simulink model "model_for_testing_errors_2"  (R2023b)
settings: Solver=VariableStepAuto  StartTime=0.0  StopTime=time_model  FixedStep=0.0001  RelTol=1e-3
values from neighbouring files (symbols this model uses):
  A_flap = [c_a, c_b, 0 ... (first row only)    [LQR_calculate.m]    (also in LQR_feedback.m; LQR_linearized_test.m; MPC_test.m; MPC_test_1.m)
  A_ind = [c_d, 0, 0 ... (first row only)    [LQR_calculate.m]    (also in LQR_feedback.m; LQR_linearized_test.m; MPC_test.m; MPC_test_1.m)
  C_drag = 0    [LQR_calculate.m]    (also in LQR_feedback.m = C_drag_arr(i); LQR_linearized_test.m = C_drag_arr(i); MPC_test.m = C_drag_arr(i); MPC_test_1.m = C_drag_arr(i))
  demp = 0    [LQR_feedback.m]    (also in LQR_linearized_test.m; MPC_params.m; MPC_test_1.m; initQuadrotorData.m)
  forward_1 = 20    [LQR_feedback.m]    (also in LQR_linearized_test.m; MPC_test_1.m)
  forward_2 = 20    [LQR_feedback.m]    (also in LQR_linearized_test.m; MPC_test_1.m)
  g = 9.81    [LQR_calculate.m]    (also in LQR_feedback.m = 9.8; LQR_linearized_test.m = 9.8; LQR_testing_gpt.m; MPC_params.m = 9.8)
  Im = 0.0135^2*0.045/2    (= 4.100625e-06)    [LQR_calculate.m]    (also in LQR_feedback.m; LQR_linearized_test.m; MPC_params.m; MPC_test.m)
  Ix = m/3*a^2/12+2*0.045*l^2    (= 0.00211347222222)    [LQR_calculate.m]    (also in LQR_feedback.m; LQR_linearized_test.m; LQR_testing_gpt.m = 0.0081; MPC_params.m)
  Iy = m/3*a^2/12+4*0.045*l^2    (= 0.00413847222222)    [LQR_calculate.m]    (also in LQR_feedback.m = 0.00211347222222; LQR_linearized_test.m = 0.00211347222222; LQR_testing_gpt.m = 0.0081; MPC_params.m = 0.00211347222222)
  Iz = m/3*a^2/4+2*0.045*l^2    (= 0.00229041666667)    [LQR_calculate.m]    (also in LQR_feedback.m = 0.00431541666667; LQR_linearized_test.m = 0.00431541666667; LQR_testing_gpt.m = 0.0142; MPC_params.m = 0.00431541666667)
  J = 2.5*10^(-6)    (= 2.5e-06)    [LQR_calculate.m]    (also in LQR_feedback.m; LQR_linearized_test.m; MPC_params.m; MPC_test.m)
  K = Y * inv(P)    [LQR_calculate.m]    (also in LQR_feedback.m = [Kx;Ky;Kz;Kphi;Ktheta;-Kpsi])
  Ke = ke    (= 0.0073)    [LQR_calculate.m]    (also in LQR_feedback.m = 0.00734; LQR_linearized_test.m = 0.00734; MPC_params.m = 0.00734; MPC_test.m)
  kf = ks*r^2*airDensity*Sblade/2    (= 1.57565625e-05)    [LQR_calculate.m]    (also in LQR_feedback.m; LQR_linearized_test.m; MPC_params.m; MPC_test.m)
  Km = kt    (= 0.0073)    [LQR_calculate.m]    (also in LQR_feedback.m = 0.00734; LQR_linearized_test.m = 0.00734; MPC_params.m = 0.00734; MPC_test.m)
  kv = 1300    [LQR_feedback.m]    (also in LQR_linearized_test.m; MPC_test_1.m; initQuadrotorData.m)
  l = 0.15    [LQR_calculate.m]    (also in LQR_feedback.m; LQR_linearized_test.m; MPC_params.m; MPC_test.m)
  L = La    (= 5e-05)    [LQR_calculate.m]    (also in LQR_feedback.m = 0.0001; LQR_linearized_test.m = 0.0001; MPC_params.m = 0.0001; MPC_test.m)
  m = size(B, 2)    [LQR_calculate.m]    (also in LQR_feedback.m = 0.65; LQR_linearized_test.m = 0.65; LQR_testing_gpt.m = 1; MPC_params.m = 0.65)
  Mode = 3    [LQR_feedback.m]    (also in LQR_linearized_test.m; MPC_test_1.m = 1)
  phi0 = 0    [LQR_feedback.m]    (also in LQR_linearized_test.m; MPC_test_1.m)
  psi0 = pi/2    (= 1.57079632679)    [LQR_feedback.m]    (also in LQR_linearized_test.m; MPC_test_1.m = 0)
  Psid = 0    [LQR_feedback.m]    (also in LQR_linearized_test.m; MPC_test_1.m)
  R = eye(4)    [LQR_calculate.m]    (also in LQR_feedback.m = 0.058; LQR_linearized_test.m = 0.058; LQR_testing_gpt.m = diag([0.1, 10, 100, 10]); MPC_params.m = 0.058)
  rho = 1.225    [LQR_calculate.m]    (also in LQR_feedback.m; LQR_linearized_test.m; MPC_params.m; MPC_test.m)
  S = l*c*4+a*b    (= 0.0169)    [LQR_calculate.m]    (also in LQR_feedback.m; LQR_linearized_test.m; MPC_params.m; MPC_test.m)
  theta0 = 0    [LQR_feedback.m]    (also in LQR_linearized_test.m; MPC_test_1.m)
  time_model = time_model_arr(i)    [LQR_feedback.m]    (also in LQR_linearized_test.m; MPC_test.m; MPC_test_1.m; plot_model_out.m)
  total_time = 60    [LQR_feedback.m]    (also in LQR_linearized_test.m; MPC_test_1.m)
  up_down = 5    [LQR_feedback.m]    (also in LQR_linearized_test.m; MPC_test_1.m)
  x0 = 0    [LQR_feedback.m]    (also in LQR_linearized_test.m; MPC_test_1.m; init_nmpc.m = zeros(nx,1))
  Xd = [Simulation.trajectory.Data(1,:)',Simulation.trajectory.Data(2,:)',Simulation.trajectory.Data(3,:)',Simulation.trajectory.Data(9,:)']    [LQR_feedback.m]    (also in LQR_linearized_test.m; MPC_test_1.m; plot_model_out.m)
  y0 = 0    [LQR_feedback.m]    (also in LQR_linearized_test.m; MPC_test_1.m)
  Yd = 0    [LQR_feedback.m]    (also in LQR_linearized_test.m; MPC_test_1.m)
  z0 = 0    [LQR_feedback.m]    (also in LQR_linearized_test.m; MPC_test_1.m)
  Zd = 0    [LQR_feedback.m]    (also in LQR_linearized_test.m; MPC_test_1.m)
libraries: sharedtransform x1
(part 1 of 2)
settings Model: Creator=Degra  LastModifiedBy=Degra

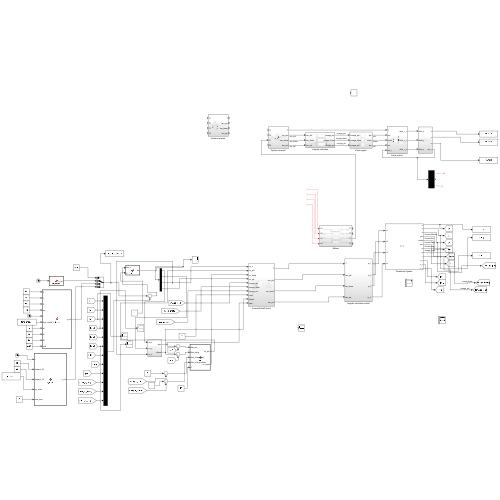
[thumbnail: Simulink's stored preview of the top-level diagram]
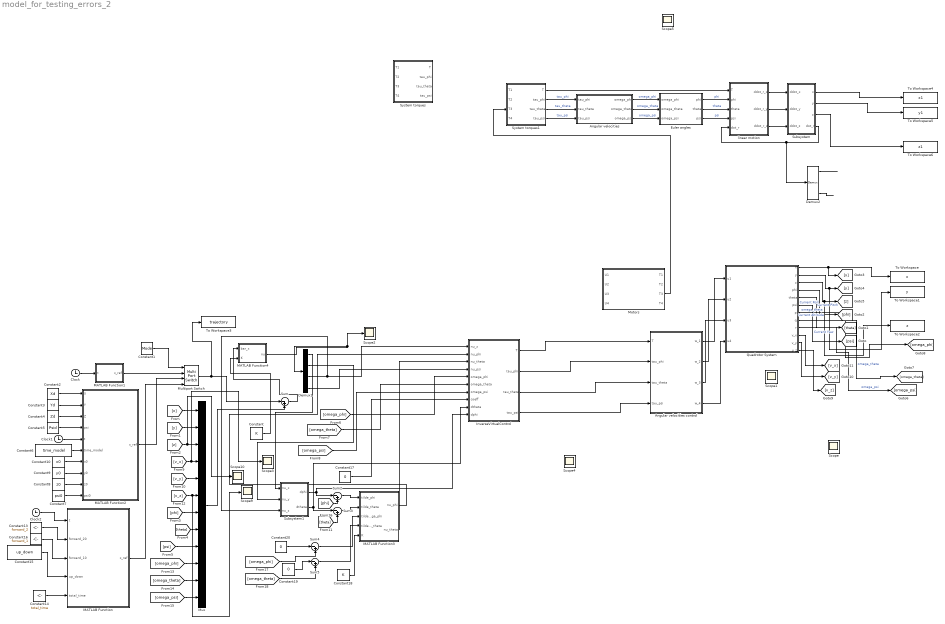
== system model_for_testing_errors_2 ==
  Angular velocities : Subsystem
  Angular velocities control : Subsystem
  Clock : Clock
  Clock1 : Clock
  Clock2 : Clock
  Constant : Constant  Value=K
  Constant1 : Constant  Value=Mode
  Constant10 : Constant  Value=x0
  Constant13 : Constant  Value=forward_2
  Constant14 : Constant  Value=total_time
  Constant15 : Constant  Value=up_down
  Constant16 : Constant  Value=forward_1
  Constant17 : Constant  Value=0
  Constant18 : Constant  Value=K
  Constant19 : Constant  Value=0
  Constant2 : Constant  Value=Xd
  Constant20 : Constant  Value=0
  Constant3 : Constant  Value=Yd
  Constant4 : Constant  Value=Zd
  Constant5 : Constant  Value=Psid
  Constant6 : Constant  Value=time_model
  Constant7 : Constant  Value=psi0
  Constant8 : Constant  Value=z0
  Constant9 : Constant  Value=y0
  Demux1 : Demux
  Demux2 : Demux  Outputs=3
  Euler angles : Subsystem
  InverseVirtualControl : Subsystem
  MATLAB Function : MATLAB Function  TreatAsAtomicUnit=on
  MATLAB Function1 : MATLAB Function  TreatAsAtomicUnit=on
  MATLAB Function2 : MATLAB Function  TreatAsAtomicUnit=on
  MATLAB Function3 : MATLAB Function  TreatAsAtomicUnit=on
  MATLAB Function4 : MATLAB Function  TreatAsAtomicUnit=on
  Motors : Subsystem
  Multiport Switch : MultiPortSwitch  SaturateOnIntegerOverflow=off  InputSameDT=off
  Mux : Mux  Inputs=12
  Quadrotor System : Subsystem
      mask Display: image('C:\Users\angel\OneDrive - Universidad Politécnica de Yucatán\CIMAT\1st semester\Robotic Systems Modeling and Control\Project\Quadrotor\images\quadrotor.jpg');
  Scope : Scope  NumInputPorts=4
  Scope1 : Scope  NumInputPorts=4
  Scope{2..5,9..10} (6 alike) : Scope
  Subsystem : Subsystem
  Subsystem1 : Subsystem
  Sum{,2..5} (5 alike) : Sum  Inputs=|-+
  System torques : Subsystem
  System torques1 : Subsystem
  To Workspace : ToWorkspace  VariableName=x  SaveFormat=Timeseries  SampleTime=-1
  To Workspace1 : ToWorkspace  VariableName=y  SaveFormat=Timeseries  SampleTime=-1
  To Workspace2 : ToWorkspace  VariableName=z  SaveFormat=Timeseries  SampleTime=-1
  To Workspace3 : ToWorkspace  VariableName=trajectory  SaveFormat=Timeseries  SampleTime=-1
  To Workspace4 : ToWorkspace  VariableName=x1  SaveFormat=Timeseries  SampleTime=-1
  To Workspace5 : ToWorkspace  VariableName=y1  SaveFormat=Timeseries  SampleTime=-1
  To Workspace6 : ToWorkspace  VariableName=z1  SaveFormat=Timeseries  SampleTime=-1
  linear motion : Subsystem
  wires:
  Quadrotor System/1(x) -> To Workspace/1, [x]
  Quadrotor System/2(y) -> To Workspace1/1, [y]
  Quadrotor System/3(z) -> To Workspace2/1, [z]  "Current Altitude"
  Quadrotor System/6(psi) -> [psi]  "Current Yaw"
  Quadrotor System/5(theta) -> [theta]  "Current Pitch"
  Quadrotor System/4(phi) -> [phi]  "Current Roll"
  Quadrotor System/9(r) -> [omega_psi]  "omega_psi"
  Quadrotor System/8(q) -> [omega_theta]  "omega_theta"
  Quadrotor System/7(p) -> [omega_phi]  "omega_theta"
  Quadrotor System/10(v_x) -> [v_x]
  Quadrotor System/11(v_y) -> [v_y]
  Quadrotor System/12(v_z) -> [v_z]
  ? -> Motors/4(U4)
  ? -> Motors/3(U3)
  ? -> Motors/2(U2)
  ? -> Motors/1(U1)
  Motors/3(T3) -> System torques1/3(T3)
  Demux2/1 -> ?
  linear motion/1(ddot_r_x) -> Subsystem/1(ddot_x)
  Demux2/3 -> ?
  Angular velocities/1(omega_phi) -> Euler angles/1(omega_phi)  "omega_phi"
  linear motion/2(ddot_r_y) -> Subsystem/2(ddot_y)
  linear motion/3(ddot_r_z) -> Subsystem/3(ddot_z)
  Euler angles/2(theta) -> linear motion/3(theta)  "theta"
  Euler angles/3(psi) -> linear motion/4(psi)  "psi"
  Euler angles/1(phi) -> linear motion/2(phi)  "phi"
  Angular velocities/2(omega_theta) -> Euler angles/2(omega_theta)  "omega_theta"
  Angular velocities/3(omega_psi) -> Euler angles/3(omega_psi)  "omega_psi"
  Subsystem/4(dot_r) -> Demux2/1, linear motion/5(dot_r)
  Subsystem/2(y) -> To Workspace5/1
  Subsystem/1(x) -> To Workspace4/1
  Subsystem/3(z) -> To Workspace6/1
  System torques1/4(tau_psi) -> Angular velocities/3(tau_psi)  "tau_psi"
  System torques1/3(tau_theta) -> Angular velocities/2(tau_theta)  "tau_theta"
  System torques1/2(tau_phi) -> Angular velocities/1(tau_phi)  "tau_phi"
  System torques1/1(T) -> linear motion/1(T)
  [omega_phi] -> Sum4/2
  MATLAB Function3/2(nu_theta) -> InverseVirtualControl/3(nu_theta)
  InverseVirtualControl/1(T) -> Angular velocities control/1(T)
  Subsystem1/1(dphi) -> Sum2/1, InverseVirtualControl/10(dphi)
  Sum4/1 -> MATLAB Function3/3(tilde_omega_phi)
  MATLAB Function3/1(nu_phi) -> InverseVirtualControl/2(nu_phi)
  Sum2/1 -> MATLAB Function3/1(tilde_phi)
  Demux1/4 -> InverseVirtualControl/4(nu_psi)
  Constant18/1 -> MATLAB Function3/5(K)
  [omega_theta] -> Sum5/2
  [phi] -> Sum2/2
  Sum5/1 -> MATLAB Function3/4(tilde_omega_theta)
  [theta] -> Sum3/2
  Sum3/1 -> MATLAB Function3/2(tilde_theta)
  [omega_theta] -> InverseVirtualControl/6(omega_theta)
  [omega_psi] -> InverseVirtualControl/7(omega_psi)
  Constant1/1 -> Multiport Switch/1
  Demux1/1 -> Subsystem1/1(nu_x)
  Constant/1 -> MATLAB Function4/2(K)
  InverseVirtualControl/4(tau_psi) -> Angular velocities control/4("tau_psi ")
  MATLAB Function4/1(nu) -> Scope2/1, Demux1/1
  Constant17/1 -> InverseVirtualControl/8(coeff)
  Sum/1 -> MATLAB Function4/1(bar_x)
  [phi] -> Mux/7
  Constant9/1 -> MATLAB Function2/8(y0)
  Constant6/1 -> MATLAB Function2/6(time_model)
  [omega_phi] -> InverseVirtualControl/5(omega_phi)
  MATLAB Function2/1(x_ref) -> Multiport Switch/3
  Constant20/1 -> Sum4/1
  InverseVirtualControl/2(tau_phi) -> Angular velocities control/2(tau_phi)
  Clock1/1 -> MATLAB Function2/5(t)
  Constant7/1 -> MATLAB Function2/10(psi0)
  Clock2/1 -> MATLAB Function/1(t)
  Demux1/3 -> Subsystem1/3(nu_z), InverseVirtualControl/1(nu_z)
  Constant19/1 -> Sum5/1
  [omega_theta] -> Mux/11
  Constant15/1 -> MATLAB Function/4(up_down)
  Constant16/1 -> MATLAB Function/3(forward_10)
  Constant13/1 -> MATLAB Function/2(forward_20)
  Subsystem1/2(dtheta) -> Sum3/1, InverseVirtualControl/9(dtheta)
  MATLAB Function1/1(x_ref) -> Multiport Switch/2
  Constant14/1 -> MATLAB Function/5(total_time)
  Mux/1 -> Sum/2
  Constant10/1 -> MATLAB Function2/7(x0)
  [omega_psi] -> Mux/12
  [y] -> Mux/2
  [v_z] -> Scope9/1, Mux/6
  InverseVirtualControl/3(tau_theta) -> Angular velocities control/3(tau_theta)
  Constant3/1 -> MATLAB Function2/2(Y)
  Constant4/1 -> MATLAB Function2/3(Z)
  [v_x] -> Scope3/1, Mux/4
  [v_y] -> Mux/5
  [omega_phi] -> Mux/10
  [z] -> Scope10/1, Mux/3
  [psi] -> Mux/9
  Constant8/1 -> MATLAB Function2/9(z0)
  [x] -> Mux/1
  [theta] -> Mux/8
  Clock/1 -> MATLAB Function1/1(t)
  MATLAB Function/1(x_ref) -> Multiport Switch/4
  Constant2/1 -> MATLAB Function2/1(X)
  Multiport Switch/1 -> Sum/1, To Workspace3/1
  Constant5/1 -> MATLAB Function2/4(psi)
  Angular velocities control/1(w_1) -> Quadrotor System/1(u1)
  Angular velocities control/2(w_2) -> Quadrotor System/2(u2)
  Angular velocities control/3(w_3) -> Quadrotor System/3(u3)
  Angular velocities control/4("w_4 ") -> Quadrotor System/4(u4)
  Demux1/2 -> Subsystem1/2(nu_y)

== system model_for_testing_errors_2/Angular velocities ==
  tau_phi : Inport
  tau_theta : Inport  Port=2
  tau_psi : Inport  Port=3
  Subsystem1 : Subsystem
  Subsystem2 : Subsystem
  Subsystem3 : Subsystem
  omega_phi : Outport
  omega_theta : Outport  Port=2
  omega_psi : Outport  Port=3
  wires:
  Subsystem2/1(omega_theta) -> omega_theta/1, Subsystem1/2(omega_theta), Subsystem3/3(omega_theta)  "omega_theta"
  tau_theta/1 -> Subsystem2/1(tau_theta)
  Subsystem1/1(omega_phi) -> omega_phi/1, Subsystem3/2(omega_phi), Subsystem2/2(omega_phi)  "omega_phi"
  Subsystem3/1(omega_psi) -> omega_psi/1, Subsystem2/3(omega_psi), Subsystem1/3(omega_psi)  "omega_psi"
  tau_phi/1 -> Subsystem1/1(tau_phi)
  tau_psi/1 -> Subsystem3/1(tau_psi)

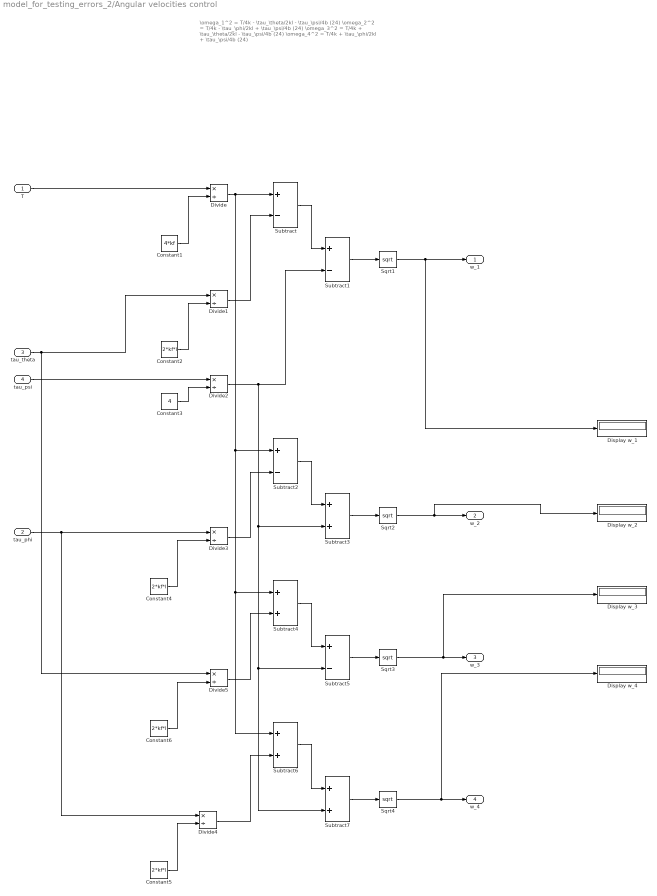
== system model_for_testing_errors_2/Angular velocities control ==
  note: \omega_1^2 = T/4k - \tau_\theta/2kl - \tau_\psi/4b   (24)
      |
      | \omega_2^2 = T/4k - \tau_\phi/2kl + \tau_\psi/4b   (24)
      |
      | \omega_3^2 = T/4k + \tau_\theta/2kl - \tau_\psi/4b   (24)
      |
      | \omega_4^2 = T/4k + \tau_\phi/2kl + \tau_\psi/4b   (24)
  T : Inport
  tau_phi : Inport  Port=2
  tau_theta : Inport  Port=3
  "tau_psi " : Inport  Port=4
  Constant1 : Constant  Value=4*kf
  Constant{2,4..6} (4 alike) : Constant  Value=2*kf*l
  Constant3 : Constant  Value=4
  Display w_{1..4} (4 alike) : Display
  Divide{,1..5} (6 alike) : Product  Inputs=*/
  Sqrt1 : Sqrt
  Sqrt2 : Sqrt  OutputSignalType=real
  Sqrt3 : Sqrt
  Sqrt4 : Sqrt
  Subtract{,1..2,5} (4 alike) : Sum  Inputs=+-
  Subtract{3..4,6..7} (4 alike) : Sum
  w_1 : Outport
  w_2 : Outport  Port=2
  w_3 : Outport  Port=3
  "w_4 " : Outport  Port=4
  wires:
  Constant1/1 -> Divide/2
  T/1 -> Divide/1
  Divide/1 -> Subtract4/1, Subtract6/1, Subtract2/1, Subtract/1
  Constant2/1 -> Divide1/2
  tau_theta/1 -> Divide5/1, Divide1/1
  Divide1/1 -> Subtract/2
  Subtract/1 -> Subtract1/1
  Constant3/1 -> Divide2/2
  Subtract1/1 -> Sqrt1/1
  Sqrt1/1 -> Display w_1/1, w_1/1
  Constant4/1 -> Divide3/2
  tau_phi/1 -> Divide4/1, Divide3/1
  Divide3/1 -> Subtract2/2
  Subtract2/1 -> Subtract3/1
  "tau_psi "/1 -> Divide2/1
  Divide2/1 -> Subtract7/2, Subtract5/2, Subtract3/2, Subtract1/2
  Sqrt2/1 -> Display w_2/1, w_2/1
  Subtract3/1 -> Sqrt2/1
  Constant6/1 -> Divide5/2
  Divide5/1 -> Subtract4/2
  Subtract5/1 -> Sqrt3/1
  Subtract4/1 -> Subtract5/1
  Sqrt3/1 -> Display w_3/1, w_3/1
  Subtract7/1 -> Sqrt4/1
  Constant5/1 -> Divide4/2
  Divide4/1 -> Subtract6/2
  Subtract6/1 -> Subtract7/1
  Sqrt4/1 -> Display w_4/1, "w_4 "/1

== system model_for_testing_errors_2/Euler angles ==
  omega_phi : Inport
  omega_theta : Inport  Port=2
  omega_psi : Inport  Port=3
  Subsystem1 : Subsystem
  Subsystem2 : Subsystem
  Subsystem3 : Subsystem
  phi : Outport
  theta : Outport  Port=2
  psi : Outport  Port=3
  wires:
  Subsystem2/1(theta) -> theta/1, Subsystem1/2(theta), Subsystem3/4(theta)  "theta"
  Subsystem1/1(phi) -> phi/1, Subsystem3/1(phi), Subsystem2/1(phi)  "phi"
  omega_theta/1 -> Subsystem3/2(omega_theta), Subsystem1/3(omega_theta), Subsystem2/2(omega_theta)
  omega_psi/1 -> Subsystem2/3(omega_psi), Subsystem3/3(omega_psi), Subsystem1/4(omega_psi)
  omega_phi/1 -> Subsystem1/1(omega_phi)
  Subsystem3/1(psi) -> psi/1  "psi"

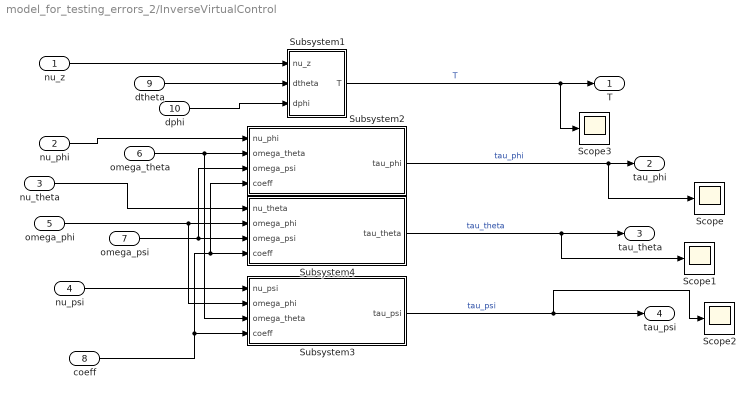
== system model_for_testing_errors_2/InverseVirtualControl ==
  nu_z : Inport
  nu_phi : Inport  Port=2
  nu_theta : Inport  Port=3
  nu_psi : Inport  Port=4
  omega_phi : Inport  Port=5
  omega_theta : Inport  Port=6
  omega_psi : Inport  Port=7
  coeff : Inport  Port=8
  dtheta : Inport  Port=9
  dphi : Inport  Port=10
  Scope{,1..3} (4 alike) : Scope
  Subsystem1 : Subsystem
  Subsystem2 : Subsystem
  Subsystem3 : Subsystem
  Subsystem4 : Subsystem
  T : Outport
  tau_phi : Outport  Port=2
  tau_theta : Outport  Port=3
  tau_psi : Outport  Port=4
  wires:
  nu_psi/1 -> Subsystem3/1(nu_psi)
  omega_psi/1 -> Subsystem2/3(omega_psi), Subsystem4/3(omega_psi)
  omega_theta/1 -> Subsystem3/3(omega_theta), Subsystem2/2(omega_theta)
  nu_phi/1 -> Subsystem2/1(nu_phi)
  omega_phi/1 -> Subsystem3/2(omega_phi), Subsystem4/2(omega_phi)
  coeff/1 -> Subsystem2/4(coeff), Subsystem4/4(coeff), Subsystem3/4(coeff)
  nu_z/1 -> Subsystem1/1(nu_z)
  Subsystem2/1(tau_phi) -> Scope/1, tau_phi/1  "tau_phi"
  nu_theta/1 -> Subsystem4/1(nu_theta)
  Subsystem1/1(T) -> Scope3/1, T/1  "T"
  Subsystem4/1(tau_theta) -> Scope1/1, tau_theta/1  "tau_theta"
  Subsystem3/1(tau_psi) -> Scope2/1, tau_psi/1  "tau_psi"
  dtheta/1 -> Subsystem1/2(dtheta)
  dphi/1 -> Subsystem1/3(dphi)

== system model_for_testing_errors_2/Motors ==
  U1 : Inport
  U2 : Inport  Port=2
  U3 : Inport  Port=3
  U4 : Inport  Port=4
  Gain{,1..3} (4 alike) : Gain  Gain=kv
  Subsystem : Subsystem  Commented=on
  Subsystem1 : Subsystem  Commented=on
  Subsystem2 : Subsystem  Commented=on
  Subsystem3 : Subsystem  Commented=on
  T1 : Outport
  T2 : Outport  Port=2
  T3 : Outport  Port=3
  T4 : Outport  Port=4
  wires:
  U4/1 -> Gain3/1, Subsystem3/1(U1)
  U1/1 -> Gain/1, Subsystem/1(U1)
  U3/1 -> Gain2/1, Subsystem2/1(U1)
  U2/1 -> Gain1/1, Subsystem1/1(U1)
  Gain/1 -> T1/1
  Gain1/1 -> T2/1
  Gain2/1 -> T3/1
  Gain3/1 -> T4/1

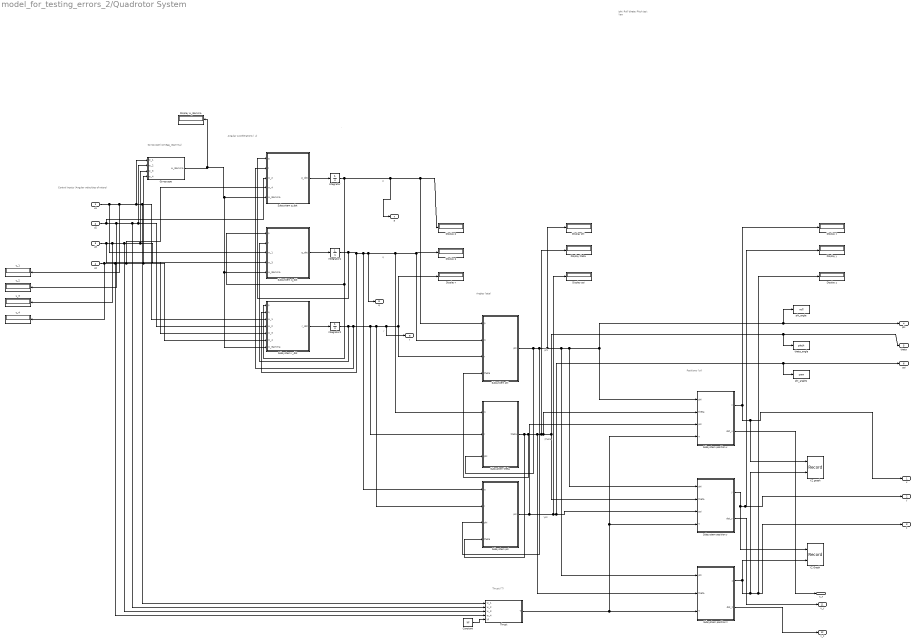
== system model_for_testing_errors_2/Quadrotor System ==
  note: Angular Accelerations (\nu)
  note: .
  note: \phi: Roll
      | \theta: Pitch
      | \psi: Yaw
  note: Control Inputs
      | (Angular velocities of rotors)
  note: Positions (\xi)
  note: Angles (\eta)
  note: Gyroscope (\omega_\Gamma)
  note: Thrust (T)
  note: p
  note: q
  note: r
  note: \phi
  note: \theta
  note: \psi
  u1 : Inport
  u2 : Inport  Port=2
  u3 : Inport  Port=3
  u4 : Inport  Port=4
  Constant : Constant  Value=kf
  Display p : Display
  Display phi : Display
  Display psi : Display
  Display q : Display
  Display r : Display
  Display theta : Display
  Display w_Gamma : Display
  Display x : Display
  Display y : Display
  Display z : Display
  Gyroscope : MATLAB Function  TreatAsAtomicUnit=on
  Integrator : Integrator
  Integrator1 : Integrator
  Integrator2 : Integrator
  Subsystem p_dot : Subsystem
  Subsystem phi : Subsystem
  Subsystem position x : Subsystem
  Subsystem position y : Subsystem
  Subsystem position z : Subsystem
  Subsystem psi : Subsystem
  Subsystem q_dot : Subsystem
  Subsystem r_dot : Subsystem
  Subsystem theta : Subsystem
  Thrust : MATLAB Function  TreatAsAtomicUnit=on
  XZ graph : Record  FileSettingsInternal="{\"entries\":[{\"content\":{\"excelSettings\":{\"content\":{},\"type\":\"Streamout.ExcelSettings\"}},\"type\":\"Streamout.FileSettingStorage\",\"uuid\":\"\"}],\"packageUris\":[\"http:\\/\\/schema.mathworks.com\\/mf0\\/streamout_blocks\\/R2020a\"],\"version\":\"1.0\"}"  Layout=[1 1]  SignalsInternal="{\"entries\":[{\"content\":{\"signals\":[{\"content\":{\"blockPath\":[],\"dimensions\":[1],\"domain\":\"\",\"lineColor\":\"#77ac30\",\"port\":1,\"sid\":[\"\"],\"signalID\":19370,\"signalName\":\"Subsystem position x:1\"},\"type\":\"RecordBlkView.Signal\",\"uuid\":\"\"},{\"content\":{\"blockPath\":[],\"dimensions\":[1],\"domain\":\"\",\"lineColor\":\"#4dbeee\",\"port\":2,\"sid\":[\"\"],\"signalID\":19374,\"signalName\":\"Subsystem position z:1\"},\"type\":\"RecordBlkView.Signal\",\"uuid\":\"\"}]},\"type\":\"RecordBlkView.InputSignals\",\"uuid\":\"\"}],\"packageUris\":[\"http:\\/\\/schema.mathworks.com\\/mf0\\/streamout_blocks\\/R2020a\"],\"version\":\"1.0\"}"  VisualizationBindings="{\"xyplotplugin\":{\"info\":[{\"series\":[],\"subplotID\":1}]}}"  CompatibilityTag=XY  st=-1
  YZ Graph : Record  FileSettingsInternal="{\"entries\":[{\"content\":{\"excelSettings\":{\"content\":{},\"type\":\"Streamout.ExcelSettings\"}},\"type\":\"Streamout.FileSettingStorage\",\"uuid\":\"\"}],\"packageUris\":[\"http:\\/\\/schema.mathworks.com\\/mf0\\/streamout_blocks\\/R2020a\"],\"version\":\"1.0\"}"  Layout=[1 1]  SignalsInternal="{\"entries\":[{\"content\":{\"signals\":[{\"content\":{\"blockPath\":[],\"dimensions\":[1],\"domain\":\"\",\"lineColor\":\"#a2142f\",\"port\":1,\"sid\":[\"\"],\"signalID\":19378,\"signalName\":\"Subsystem position y:1\"},\"type\":\"RecordBlkView.Signal\",\"uuid\":\"\"},{\"content\":{\"blockPath\":[],\"dimensions\":[1],\"domain\":\"\",\"lineColor\":\"#139fff\",\"port\":2,\"sid\":[\"\"],\"signalID\":19382,\"signalName\":\"Subsystem position z:1\"},\"type\":\"RecordBlkView.Signal\",\"uuid\":\"\"}]},\"type\":\"RecordBlkView.InputSignals\",\"uuid\":\"\"}],\"packageUris\":[\"http:\\/\\/schema.mathworks.com\\/mf0\\/streamout_blocks\\/R2020a\"],\"version\":\"1.0\"}"  VisualizationBindings="{\"xyplotplugin\":{\"info\":[{\"series\":[],\"subplotID\":1}]}}"  CompatibilityTag=XY  st=-1
  phi_angle : ToWorkspace  VariableName=roll  SampleTime=-1
  phi_angle1 : ToWorkspace  VariableName=yaw  SampleTime=-1
  theta_angle : ToWorkspace  VariableName=pitch  SampleTime=-1
  u_{1..4} (4 alike) : Display
  x : Outport
  y : Outport  Port=2
  z : Outport  Port=3
  phi : Outport  Port=4
  theta : Outport  Port=5
  psi : Outport  Port=6
  p : Outport  Port=7
  q : Outport  Port=8
  r : Outport  Port=9
  v_x : Outport  Port=10
  v_y : Outport  Port=11
  v_z : Outport  Port=12
  wires:
  u1/1 -> Subsystem q_dot/3(w_1), u_1/1, Gyroscope/1(w_1), Subsystem r_dot/3(w_1), Thrust/1(w_1)
  u2/1 -> Subsystem p_dot/3(w_2), u_2/1, Gyroscope/2(w_2), Subsystem r_dot/4(w_2), Thrust/2(w_2)
  u3/1 -> Subsystem q_dot/4(w_3), Gyroscope/3(w_3), Subsystem r_dot/5(w_3), Thrust/3(w_3), u_3/1
  u4/1 -> u_4/1, Gyroscope/4(w_4), Subsystem r_dot/6(w_4), Subsystem p_dot/4(w_4), Thrust/4(w_4)
  Thrust/1(T) -> Subsystem position y/4("T "), Subsystem position x/4(T), Subsystem position z/3(T)
  Subsystem phi/1("phi ") -> Subsystem theta/3("phi "), Subsystem psi/3(phi), Display phi/1, Subsystem position z/1("phi "), Subsystem position y/1("phi "), phi_angle/1, phi/1, Subsystem position x/1("phi ")
  Subsystem psi/1(psi) -> Subsystem position x/3("psi "), Display psi/1, phi_angle1/1, psi/1, Subsystem position y/3("psi ")
  Subsystem position x/1(x) -> x/1, XZ graph/1, Display x/1
  Subsystem position z/1(z) -> XZ graph/2, z/1, Display z/1, YZ Graph/2
  Subsystem position y/1("y ") -> y/1, Display y/1, YZ Graph/1
  Gyroscope/1(w_Gamma) -> Display w_Gamma/1, Subsystem r_dot/7(w_Gamma), Subsystem q_dot/5("w_Gamma "), Subsystem p_dot/5("w_Gamma ")
  Subsystem p_dot/1(p_dot) -> Integrator/1
  Subsystem q_dot/1(q_dot) -> Integrator1/1
  Subsystem r_dot/1(r_dot) -> Integrator2/1
  Integrator/1 -> Subsystem r_dot/1("p "), Subsystem q_dot/1("p "), p/1, Display p/1, Subsystem phi/1(p)
  Integrator2/1 -> Subsystem theta/2(r), Subsystem psi/2(r), r/1, Display r/1, Subsystem phi/3(r), Subsystem p_dot/2(r), Subsystem q_dot/2(r)
  Integrator1/1 -> Subsystem p_dot/1(q), Subsystem psi/1(q), Subsystem theta/1(q), Display q/1, Subsystem phi/2(q), q/1, Subsystem r_dot/2(q)
  Subsystem theta/1(theta) -> Subsystem psi/4(theta), Subsystem phi/4(theta), Subsystem position z/2("theta "), Display theta/1, Subsystem position x/2("theta "), theta_angle/1, theta/1, Subsystem position y/2("theta ")
  Subsystem position x/2(dot_x) -> v_x/1
  Subsystem position y/2(dot_y) -> v_y/1
  Subsystem position z/2(dot_z) -> v_z/1
  Constant/1 -> Thrust/5(kf)

== system model_for_testing_errors_2/Subsystem ==
  ddot_x : Inport
  ddot_y : Inport  Port=2
  ddot_z : Inport  Port=3
  Integrator10 : Integrator  InitialCondition=z0
  Integrator11 : Integrator
  Integrator6 : Integrator  InitialCondition=x0
  Integrator7 : Integrator
  Integrator8 : Integrator  InitialCondition=y0
  Integrator9 : Integrator
  Mux : Mux  Inputs=3
  x : Outport
  y : Outport  Port=2
  z : Outport  Port=3
  dot_r : Outport  Port=4
  wires:
  Integrator9/1 -> Mux/2, Integrator8/1
  Integrator7/1 -> Mux/1, Integrator6/1
  Integrator10/1 -> z/1  "z"
  Integrator11/1 -> Mux/3, Integrator10/1
  Integrator8/1 -> y/1  "y"
  ddot_x/1 -> Integrator7/1
  Mux/1 -> dot_r/1  "dot_r"
  Integrator6/1 -> x/1  "x"
  ddot_y/1 -> Integrator9/1
  ddot_z/1 -> Integrator11/1

== system model_for_testing_errors_2/Subsystem1 ==
  nu_x : Inport
  nu_y : Inport  Port=2
  nu_z : Inport  Port=3
  Atan : Trigonometry  Operator=atan2
  Atan1 : Trigonometry  Operator=atan2
  Constant18 : Constant  Value=g
  Constant19 : Constant  Value=g
  Scope : Scope
  Sum3 : Sum  Inputs=|++
  Sum4 : Sum  Inputs=|++
  dphi : Outport
  dtheta : Outport  Port=2
  wires:
  Sum4/1 -> Atan1/2
  Sum3/1 -> Atan/2
  Constant19/1 -> Sum4/2
  Constant18/1 -> Sum3/2
  nu_z/1 -> Sum3/1, Sum4/1
  Atan1/1 -> dtheta/1
  Atan/1 -> dphi/1, Scope/1
  nu_y/1 -> Atan1/1
  nu_x/1 -> Atan/1

== system model_for_testing_errors_2/System torques ==
  T1 : Inport
  T2 : Inport  Port=2
  T3 : Inport  Port=3
  T4 : Inport  Port=4
  Gain : Gain  Gain=l
  Gain1 : Gain  Gain=1.140e-7
  Gain3 : Gain  Gain=l
  Sum : Sum  Inputs=|-+
  Sum1 : Sum  Inputs=|-+
  Sum2 : Sum  Inputs=++--
  Sum3 : Sum  Inputs=++++
  T : Outport
  tau_phi : Outport  Port=2
  tau_theta : Outport  Port=3
  tau_psi : Outport  Port=4
  wires:
  T3/1 -> Sum2/3, Sum3/3, Sum/2
  T4/1 -> Sum3/2, Sum1/2, Sum2/1
  Sum2/1 -> Gain1/1  "tau_psi"
  T1/1 -> Sum2/4, Sum3/1, Sum/1
  Sum/1 -> Gain/1
  Sum1/1 -> Gain3/1
  Sum3/1 -> T/1  "T"
  T2/1 -> Sum2/2, Sum3/4, Sum1/1
  Gain3/1 -> tau_theta/1  "tau_theta"
  Gain/1 -> tau_phi/1  "tau_phi"
  Gain1/1 -> tau_psi/1

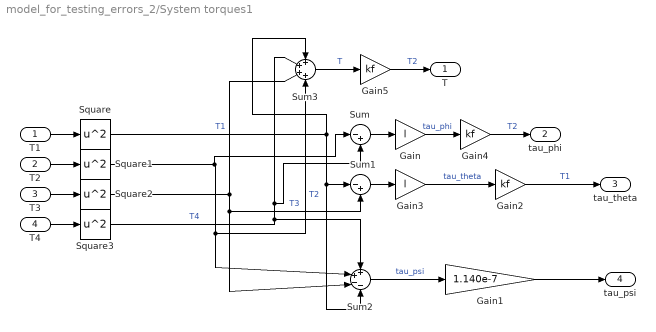
== system model_for_testing_errors_2/System torques1 ==
  T1 : Inport
  T2 : Inport  Port=2
  T3 : Inport  Port=3
  T4 : Inport  Port=4
  Gain : Gain  Gain=l
  Gain1 : Gain  Gain=1.140e-7
  Gain2 : Gain  Gain=kf
  Gain3 : Gain  Gain=l
  Gain4 : Gain  Gain=kf
  Gain5 : Gain  Gain=kf
  Square{,1..3} (4 alike) : Math  Operator=square
  Sum : Sum  Inputs=|-+
  Sum1 : Sum  Inputs=|-+
  Sum2 : Sum  Inputs=++--
  Sum3 : Sum  Inputs=++++
  T : Outport
  tau_phi : Outport  Port=2
  tau_theta : Outport  Port=3
  tau_psi : Outport  Port=4
  wires:
  T3/1 -> Square2/1
  T4/1 -> Square3/1
  Sum2/1 -> Gain1/1  "tau_psi"
  T1/1 -> Square/1
  Sum/1 -> Gain/1
  Sum1/1 -> Gain3/1
  Sum3/1 -> Gain5/1  "T"
  T2/1 -> Square1/1
  Gain3/1 -> Gain2/1  "tau_theta"
  Gain/1 -> Gain4/1  "tau_phi"
  Gain1/1 -> tau_psi/1
  Square/1 -> Sum1/1, Sum2/4, Sum3/1  "T1"
  Square1/1 -> Sum/1, Sum2/2, Sum3/4  "T2"
  Square2/1 -> Sum1/2, Sum2/3, Sum3/3  "T3"
  Square3/1 -> Sum/2, Sum3/2, Sum2/1  "T4"
  Gain4/1 -> tau_phi/1  "T2"
  Gain2/1 -> tau_theta/1  "T1"
  Gain5/1 -> T/1  "T2"

== system model_for_testing_errors_2/linear motion ==
  T : Inport
  phi : Inport  Port=2
  theta : Inport  Port=3
  psi : Inport  Port=4
  dot_r : Inport  Port=5
  Subsystem : Subsystem
  Subsystem1 : Subsystem
  Subsystem2 : Subsystem
  Subsystem3 : Subsystem
  ddot_r_x : Outport
  ddot_r_y : Outport  Port=2
  ddot_r_z : Outport  Port=3
  wires:
  T/1 -> Subsystem/1(T), Subsystem2/2(T), Subsystem3/1(T), Subsystem1/1(T)
  theta/1 -> Subsystem/2(theta), Subsystem2/3(theta), Subsystem3/4(theta), Subsystem1/3(theta)
  phi/1 -> Subsystem/3(phi), Subsystem2/4(phi), Subsystem3/2(phi), Subsystem1/2(phi)
  Subsystem1/3((F_ind+F_flap+F_drag)_z) -> Subsystem/4((F_ind+F_flap+F_drag)_z)
  psi/1 -> Subsystem3/5(psi), Subsystem2/1(psi), Subsystem1/4(psi)
  dot_r/1 -> Subsystem1/5(dot_r)
  Subsystem1/2((F_ind+F_flap+F_drag)_y) -> Subsystem2/5((F_ind+F_flap+F_drag)_y)
  Subsystem1/1((F_ind+F_flap+F_drag)_x) -> Subsystem3/3((F_ind+F_flap+F_drag)_x)
  Subsystem3/1(ddot_r_x) -> ddot_r_x/1  "ddot_r_x"
  Subsystem2/1(ddot_r_y) -> ddot_r_y/1  "ddot_r_y"
  Subsystem/1(ddot_r_z) -> ddot_r_z/1  "ddot_r_z"

== system model_for_testing_errors_2/Angular velocities/Subsystem1 ==
  tau_phi : Inport
  omega_theta : Inport  Port=2
  omega_psi : Inport  Port=3
  Gain : Gain  Gain=Iy-Iz
  Gain1 : Gain  Gain=1/Ix
  Integrator12 : Integrator
  Product : Product
  Sum : Sum  Inputs=|++
  omega_phi : Outport
  wires:
  Gain/1 -> Sum/2
  omega_theta/1 -> Product/1
  Product/1 -> Gain/1
  Sum/1 -> Gain1/1  "dot_omega_phi"
  tau_phi/1 -> Sum/1
  omega_psi/1 -> Product/2
  Gain1/1 -> Integrator12/1
  Integrator12/1 -> omega_phi/1  "omega_phi"

== system model_for_testing_errors_2/Angular velocities/Subsystem2 ==
  tau_theta : Inport
  omega_phi : Inport  Port=2
  omega_psi : Inport  Port=3
  Gain : Gain  Gain=Iz-Ix
  Gain1 : Gain  Gain=1/Iy
  Integrator12 : Integrator
  Product : Product
  Sum : Sum  Inputs=|++
  omega_theta : Outport
  wires:
  Gain/1 -> Sum/2
  Sum/1 -> Gain1/1  "omega_theta"
  omega_phi/1 -> Product/1
  Product/1 -> Gain/1
  tau_theta/1 -> Sum/1
  omega_psi/1 -> Product/2
  Gain1/1 -> Integrator12/1
  Integrator12/1 -> omega_theta/1  "omega_theta"

== system model_for_testing_errors_2/Angular velocities/Subsystem3 ==
  tau_psi : Inport
  omega_phi : Inport  Port=2
  omega_theta : Inport  Port=3
  Gain : Gain  Gain=Ix-Iy
  Gain1 : Gain  Gain=1/Iz
  Integrator12 : Integrator
  Product : Product
  Sum : Sum  Inputs=|++
  omega_psi : Outport
  wires:
  Gain/1 -> Sum/2
  omega_phi/1 -> Product/1
  Product/1 -> Gain/1
  Sum/1 -> Gain1/1  "dot_omega_psi"
  tau_psi/1 -> Sum/1
  omega_theta/1 -> Product/2
  Gain1/1 -> Integrator12/1
  Integrator12/1 -> omega_psi/1  "omega_psi"

== system model_for_testing_errors_2/Euler angles/Subsystem1 ==
  omega_phi : Inport
  theta : Inport  Port=2
  omega_theta : Inport  Port=3
  omega_psi : Inport  Port=4
  Integrator : Integrator  InitialCondition=phi0
  Product : Product
  Product1 : Product
  Product2 : Product
  Sum : Sum  Inputs=|++
  Sum1 : Sum  Inputs=|++
  Tan : Trigonometry  Operator=tan
  Tan1 : Trigonometry
  Tan2 : Trigonometry  Operator=cos
  phi : Outport
  wires:
  Product2/1 -> Sum1/2
  Tan1/1 -> Product1/2
  Sum/1 -> Integrator/1
  Sum1/1 -> Product/2
  Tan/1 -> Product/1
  Tan2/1 -> Product2/2
  Product1/1 -> Sum1/1
  omega_psi/1 -> Product2/1
  omega_theta/1 -> Product1/1
  Integrator/1 -> Tan1/1, Tan2/1, phi/1  "phi"
  theta/1 -> Tan/1
  omega_phi/1 -> Sum/1
  Product/1 -> Sum/2

== system model_for_testing_errors_2/Euler angles/Subsystem2 ==
  phi : Inport
  omega_theta : Inport  Port=2
  omega_psi : Inport  Port=3
  Integrator : Integrator  InitialCondition=theta0
  Product1 : Product
  Product2 : Product
  Sum1 : Sum  Inputs=|+-
  Tan1 : Trigonometry  Operator=cos
  Tan2 : Trigonometry
  theta : Outport
  wires:
  Product2/1 -> Sum1/2
  Tan1/1 -> Product1/2
  Tan2/1 -> Product2/2
  Product1/1 -> Sum1/1
  omega_psi/1 -> Product2/1
  Integrator/1 -> theta/1  "theta"
  phi/1 -> Tan2/1, Tan1/1
  omega_theta/1 -> Product1/1
  Sum1/1 -> Integrator/1

== system model_for_testing_errors_2/Euler angles/Subsystem3 ==
  phi : Inport
  omega_theta : Inport  Port=2
  omega_psi : Inport  Port=3
  theta : Inport  Port=4
  Divide : Product  Inputs=*/
  Divide1 : Product  Inputs=*/
  Integrator : Integrator  InitialCondition=psi0
  Product1 : Product
  Product2 : Product
  Sum1 : Sum  Inputs=|++
  Tan1 : Trigonometry
  Tan2 : Trigonometry  Operator=cos
  Tan3 : Trigonometry  Operator=cos
  Tan4 : Trigonometry  Operator=cos
  psi : Outport
  wires:
  Product2/1 -> Sum1/2
  Product1/1 -> Sum1/1
  omega_psi/1 -> Product2/1
  Integrator/1 -> psi/1  "psi"
  phi/1 -> Tan1/1, Tan2/1
  theta/1 -> Tan4/1, Tan3/1
  Divide/1 -> Product2/2
  Tan2/1 -> Divide/1
  Tan3/1 -> Divide/2
  Divide1/1 -> Product1/2
  Tan1/1 -> Divide1/1
  Tan4/1 -> Divide1/2
  omega_theta/1 -> Product1/1
  Sum1/1 -> Integrator/1

== system model_for_testing_errors_2/InverseVirtualControl/Subsystem1 ==
  nu_z : Inport
  dtheta : Inport  Port=2
  dphi : Inport  Port=3
  Constant17 : Constant  Value=g
  Cos : Trigonometry  Operator=cos
  Cos1 : Trigonometry  Operator=cos
  Divide : Product  Inputs=*/
  Gain : Gain  Gain=m
  Product : Product
  Scope{,1..3} (4 alike) : Scope
  Sum2 : Sum  Inputs=++|
  T : Outport
  wires:
  nu_z/1 -> Sum2/1, Scope/1
  Cos/1 -> Product/1
  Constant17/1 -> Sum2/2
  Product/1 -> Scope2/1, Divide/2
  Sum2/1 -> Gain/1
  Cos1/1 -> Product/2
  Divide/1 -> Scope3/1, T/1  "T"
  Gain/1 -> Scope1/1, Divide/1
  dtheta/1 -> Cos/1
  dphi/1 -> Cos1/1

== system model_for_testing_errors_2/InverseVirtualControl/Subsystem2 ==
  nu_phi : Inport
  omega_theta : Inport  Port=2
  omega_psi : Inport  Port=3
  coeff : Inport  Port=4
  Gain : Gain  Gain=Iy-Iz
  Gain1 : Gain  Gain=Ix
  Product : Product  Inputs=3
  Sum2 : Sum  Inputs=+-
  tau_phi : Outport
  wires:
  omega_theta/1 -> Product/1
  Gain1/1 -> Sum2/1
  nu_phi/1 -> Gain1/1
  coeff/1 -> Product/3
  Product/1 -> Gain/1
  Sum2/1 -> tau_phi/1  "tau_phi"
  Gain/1 -> Sum2/2
  omega_psi/1 -> Product/2

== system model_for_testing_errors_2/InverseVirtualControl/Subsystem3 ==
  nu_psi : Inport
  omega_phi : Inport  Port=2
  omega_theta : Inport  Port=3
  coeff : Inport  Port=4
  Gain : Gain  Gain=Ix-Iy
  Gain1 : Gain  Gain=Iz
  Product : Product  Inputs=3
  Sum2 : Sum  Inputs=+-
  tau_psi : Outport
  wires:
  omega_phi/1 -> Product/1
  Gain1/1 -> Sum2/1
  nu_psi/1 -> Gain1/1
  coeff/1 -> Product/3
  Product/1 -> Gain/1
  Sum2/1 -> tau_psi/1  "tau_psi"
  Gain/1 -> Sum2/2
  omega_theta/1 -> Product/2

== system model_for_testing_errors_2/InverseVirtualControl/Subsystem4 ==
  nu_theta : Inport
  omega_phi : Inport  Port=2
  omega_psi : Inport  Port=3
  coeff : Inport  Port=4
  Gain : Gain  Gain=Iz-Ix
  Gain1 : Gain  Gain=Iy
  Product : Product  Inputs=3
  Sum2 : Sum  Inputs=+-
  tau_theta : Outport
  wires:
  omega_phi/1 -> Product/1
  Gain1/1 -> Sum2/1
  nu_theta/1 -> Gain1/1
  coeff/1 -> Product/3
  Product/1 -> Gain/1
  Sum2/1 -> tau_theta/1  "tau_theta"
  Gain/1 -> Sum2/2
  omega_psi/1 -> Product/2

== system model_for_testing_errors_2/Motors/Subsystem ==
  U1 : Inport
  Add : Sum  Inputs=+--
  Add1 : Sum  Inputs=+-
  Gain : Gain  Gain=demp
  Gain1 : Gain  Gain=Km
  Gain2 : Gain  Gain=1/L
  Gain3 : Gain  Gain=Ke
  Gain5 : Gain  Gain=R
  Gain6 : Gain  Gain=1/J
  Integrator : Integrator
  Integrator1 : Integrator
  T1 : Outport
  wires:
  Gain2/1 -> Integrator/1
  Add/1 -> Gain2/1
  Integrator/1 -> Gain1/1, Gain5/1
  Gain5/1 -> Add/3
  U1/1 -> Add/1
  Gain1/1 -> Add1/1
  Add1/1 -> Gain6/1
  Integrator1/1 -> T1/1, Gain3/1, Gain/1
  Gain3/1 -> Add/2
  Gain/1 -> Add1/2
  Gain6/1 -> Integrator1/1

== system model_for_testing_errors_2/Motors/Subsystem1 ==
  U1 : Inport
  Add : Sum  Inputs=+--
  Add1 : Sum  Inputs=+-
  Gain : Gain  Gain=demp
  Gain1 : Gain  Gain=Km
  Gain2 : Gain  Gain=1/L
  Gain3 : Gain  Gain=Ke
  Gain5 : Gain  Gain=R
  Gain6 : Gain  Gain=1/J
  Integrator : Integrator
  Integrator1 : Integrator
  T1 : Outport
  wires:
  Gain2/1 -> Integrator/1
  Add/1 -> Gain2/1
  Integrator/1 -> Gain1/1, Gain5/1
  Gain5/1 -> Add/3
  U1/1 -> Add/1
  Gain1/1 -> Add1/1
  Add1/1 -> Gain6/1
  Integrator1/1 -> T1/1, Gain3/1, Gain/1
  Gain3/1 -> Add/2
  Gain/1 -> Add1/2
  Gain6/1 -> Integrator1/1

== system model_for_testing_errors_2/Motors/Subsystem2 ==
  U1 : Inport
  Add : Sum  Inputs=+--
  Add1 : Sum  Inputs=+-
  Gain : Gain  Gain=demp
  Gain1 : Gain  Gain=Km
  Gain2 : Gain  Gain=1/L
  Gain3 : Gain  Gain=Ke
  Gain5 : Gain  Gain=R
  Gain6 : Gain  Gain=1/J
  Integrator : Integrator
  Integrator1 : Integrator
  T1 : Outport
  wires:
  Gain2/1 -> Integrator/1
  Add/1 -> Gain2/1
  Integrator/1 -> Gain1/1, Gain5/1
  Gain5/1 -> Add/3
  U1/1 -> Add/1
  Gain1/1 -> Add1/1
  Add1/1 -> Gain6/1
  Integrator1/1 -> T1/1, Gain3/1, Gain/1
  Gain3/1 -> Add/2
  Gain/1 -> Add1/2
  Gain6/1 -> Integrator1/1

== system model_for_testing_errors_2/Motors/Subsystem3 ==
  U1 : Inport
  Add : Sum  Inputs=+--
  Add1 : Sum  Inputs=+-
  Gain : Gain  Gain=demp
  Gain1 : Gain  Gain=Km
  Gain2 : Gain  Gain=1/L
  Gain3 : Gain  Gain=Ke
  Gain5 : Gain  Gain=R
  Gain6 : Gain  Gain=1/J
  Integrator : Integrator
  Integrator1 : Integrator
  T1 : Outport
  wires:
  Gain2/1 -> Integrator/1
  Add/1 -> Gain2/1
  Integrator/1 -> Gain1/1, Gain5/1
  Gain5/1 -> Add/3
  U1/1 -> Add/1
  Gain1/1 -> Add1/1
  Add1/1 -> Gain6/1
  Integrator1/1 -> T1/1, Gain3/1, Gain/1
  Gain3/1 -> Add/2
  Gain/1 -> Add1/2
  Gain6/1 -> Integrator1/1

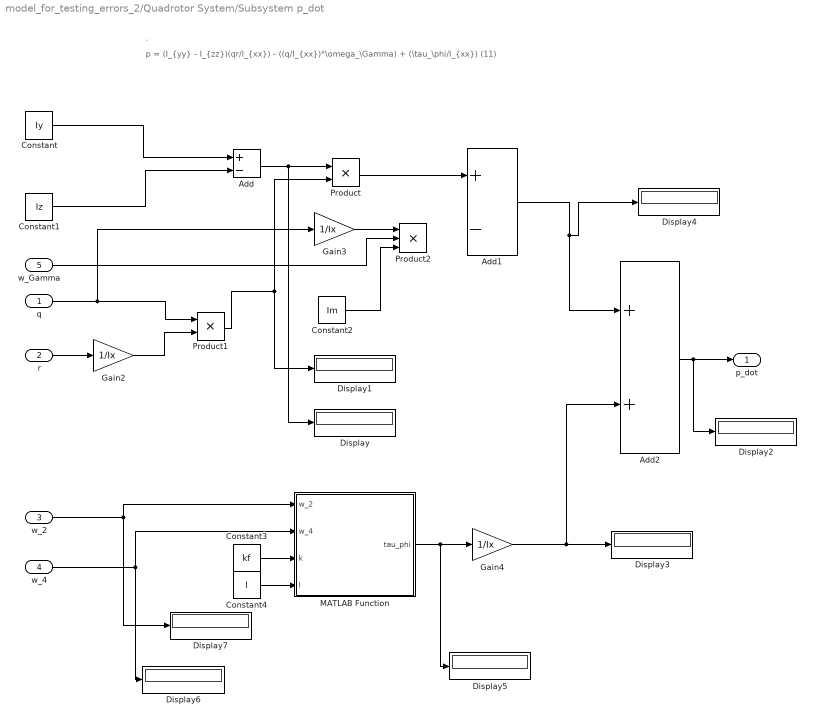
== system model_for_testing_errors_2/Quadrotor System/Subsystem p_dot ==
  note: p = (I_{yy} - I_{zz})(qr/I_{xx}) - ((q/I_{xx})*\omega_\Gamma) + (\tau_\phi/I_{xx}) (11)
  note: .
  q : Inport
  r : Inport  Port=2
  w_2 : Inport  Port=3
  w_4 : Inport  Port=4
  "w_Gamma " : Inport  Port=5
  Add : Sum  Inputs=+-
  Add1 : Sum  Inputs=+-
  Add2 : Sum
  Constant : Constant  Value=Iy
  Constant1 : Constant  Value=Iz
  Constant2 : Constant  Value=Im
  Constant3 : Constant  Value=kf
  Constant4 : Constant  Value=l
  Display{,1..7} (8 alike) : Display
  Gain2 : Gain  Gain=1/Ix
  Gain3 : Gain  Gain=1/Ix
  Gain4 : Gain  Gain=1/Ix
  MATLAB Function : MATLAB Function  TreatAsAtomicUnit=on
  Product : Product
  Product1 : Product
  Product2 : Product  Inputs=3
  p_dot : Outport
  wires:
  Constant/1 -> Add/1
  Constant1/1 -> Add/2
  Add/1 -> Display/1, Product/1
  Product/1 -> Add1/1
  Add2/1 -> p_dot/1, Display2/1
  r/1 -> Gain2/1
  Gain2/1 -> Product1/2
  q/1 -> Gain3/1, Product1/1
  Gain3/1 -> Product2/1
  Product1/1 -> Display1/1, Product/2
  MATLAB Function/1(tau_phi) -> Display5/1, Gain4/1
  w_2/1 -> MATLAB Function/1(w_2), Display7/1
  w_4/1 -> Display6/1, MATLAB Function/2(w_4)
  "w_Gamma "/1 -> Product2/2
  Gain4/1 -> Display3/1, Add2/2
  Add1/1 -> Display4/1, Add2/1
  Constant2/1 -> Product2/3
  Constant3/1 -> MATLAB Function/3(k)
  Constant4/1 -> MATLAB Function/4(l)

== system model_for_testing_errors_2/Quadrotor System/Subsystem phi ==
  note: \phi
  note: \phi
  note: .
  note: \phi = p + q(S_\phiT_\theta) + r(C_\phiT_\theta) (4)
  note: .
  p : Inport
  q : Inport  Port=2
  r : Inport  Port=3
  theta : Inport  Port=4
  Display1 : Display
  Display10 : Display
  Display9 : Display
  Integrator6 : Integrator  InitialConditionSource=external  InitialCondition=-0.1
  Product5 : Product  Inputs=3
  Product6 : Product  Inputs=3
  Roll Initial : Constant  Value=0
  Z''3 : Sum  Inputs=+++
  "cos " : Trigonometry  Operator=cos
  cos 1 : Trigonometry
  tan 1 : Trigonometry  Operator=tan
  tan 5 : Trigonometry  Operator=tan
  "phi " : Outport
  wires:
  "cos "/1 -> Product5/1
  Product5/1 -> Display10/1, Z''3/1
  theta/1 -> tan 5/1, tan 1/1
  Integrator6/1 -> "cos "/1, Display1/1, cos 1/1, "phi "/1
  tan 5/1 -> Product5/3
  Z''3/1 -> Integrator6/1
  q/1 -> Product6/2
  Product6/1 -> Display9/1, Z''3/3
  p/1 -> Z''3/2
  cos 1/1 -> Product6/1
  tan 1/1 -> Product6/3
  r/1 -> Product5/2
  Roll Initial/1 -> Integrator6/2

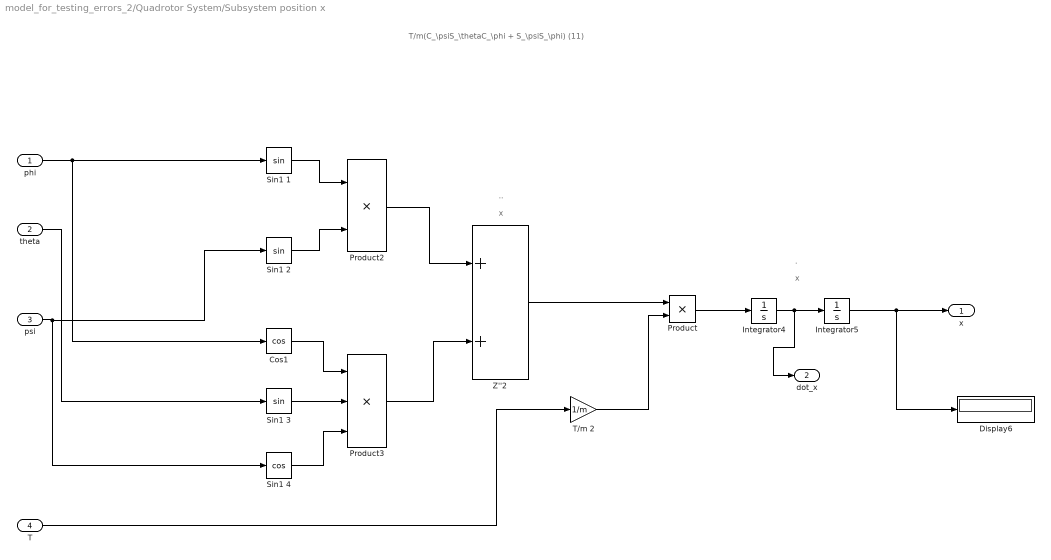
== system model_for_testing_errors_2/Quadrotor System/Subsystem position x ==
  note: ..
  note: x
  note: .
  note: x
  note: T/m(C_\psiS_\thetaC_\phi + S_\psiS_\phi) (11)
  "phi " : Inport
  "theta " : Inport  Port=2
  "psi " : Inport  Port=3
  T : Inport  Port=4
  Cos1 : Trigonometry  Operator=cos
  Display6 : Display
  Integrator4 : Integrator
  Integrator5 : Integrator
  Product : Product
  Product2 : Product
  Product3 : Product  Inputs=3
  Sin1 1 : Trigonometry
  Sin1 2 : Trigonometry
  Sin1 3 : Trigonometry
  Sin1 4 : Trigonometry  Operator=cos
  T/m 2 : Gain  Gain=1/m
  Z''2 : Sum
  x : Outport
  dot_x : Outport  Port=2
  wires:
  "phi "/1 -> Cos1/1, Sin1 1/1
  "psi "/1 -> Sin1 2/1, Sin1 4/1
  Integrator4/1 -> dot_x/1, Integrator5/1
  Product2/1 -> Z''2/1
  Product3/1 -> Z''2/2
  "theta "/1 -> Sin1 3/1
  Sin1 1/1 -> Product2/1
  Sin1 3/1 -> Product3/2
  Sin1 2/1 -> Product2/2
  Sin1 4/1 -> Product3/3
  Cos1/1 -> Product3/1
  Integrator5/1 -> x/1, Display6/1
  T/m 2/1 -> Product/2
  T/1 -> T/m 2/1
  Z''2/1 -> Product/1
  Product/1 -> Integrator4/1

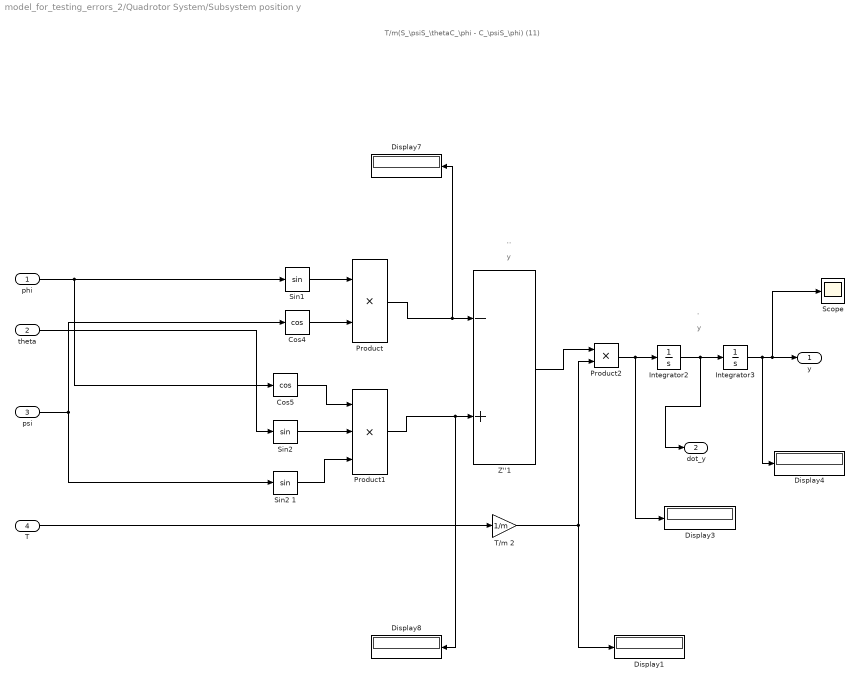
== system model_for_testing_errors_2/Quadrotor System/Subsystem position y ==
  note: T/m(S_\psiS_\thetaC_\phi - C_\psiS_\phi) (11)
  note: ..
  note: y
  note: y
  note: .
  "phi " : Inport
  "theta " : Inport  Port=2
  "psi " : Inport  Port=3
  "T " : Inport  Port=4
  Cos4 : Trigonometry  Operator=cos
  Cos5 : Trigonometry  Operator=cos
  Display{1,3..4,7..8} (5 alike) : Display
  Integrator2 : Integrator
  Integrator3 : Integrator
  Product : Product
  Product1 : Product  Inputs=3
  Product2 : Product
  Scope : Scope
  "Sin1 " : Trigonometry
  "Sin2 " : Trigonometry
  Sin2 1 : Trigonometry
  T/m 2 : Gain  Gain=1/m
  Z''1 : Sum  Inputs=-+
  "y " : Outport
  dot_y : Outport  Port=2
  wires:
  Integrator2/1 -> dot_y/1, Integrator3/1
  "theta "/1 -> "Sin2 "/1
  Integrator3/1 -> "y "/1, Scope/1, Display4/1
  "phi "/1 -> "Sin1 "/1, Cos5/1
  Product/1 -> Display7/1, Z''1/1
  Cos4/1 -> Product/2
  "psi "/1 -> Cos4/1, Sin2 1/1
  Sin2 1/1 -> Product1/3
  Product1/1 -> Display8/1, Z''1/2
  Cos5/1 -> Product1/1
  "Sin2 "/1 -> Product1/2
  "Sin1 "/1 -> Product/1
  "T "/1 -> T/m 2/1
  Z''1/1 -> Product2/1
  T/m 2/1 -> Display1/1, Product2/2
  Product2/1 -> Display3/1, Integrator2/1

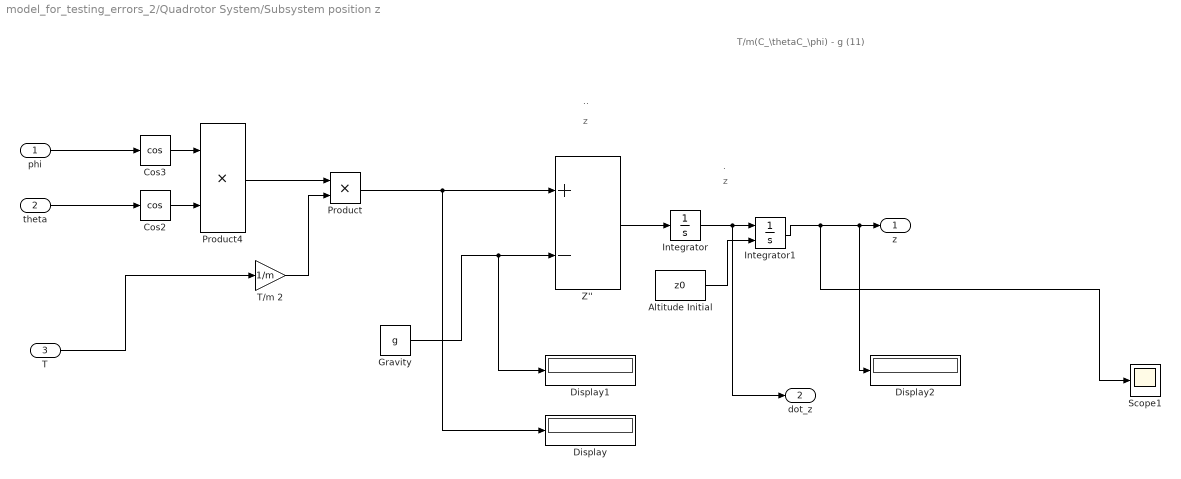
== system model_for_testing_errors_2/Quadrotor System/Subsystem position z ==
  note: z
  note: ..
  note: .
  note: z
  note: T/m(C_\thetaC_\phi) - g (11)
  "phi " : Inport
  "theta " : Inport  Port=2
  T : Inport  Port=3
  Altitude Initial : Constant  Value=z0
  Cos2 : Trigonometry  Operator=cos
  Cos3 : Trigonometry  Operator=cos
  Display : Display
  Display1 : Display
  Display2 : Display
  Gravity : Constant  Value=g
  Integrator : Integrator
  Integrator1 : Integrator  InitialConditionSource=external
  Product : Product
  Product4 : Product
  Scope1 : Scope
  T/m 2 : Gain  Gain=1/m
  Z'' : Sum  Inputs=+-
  z : Outport
  dot_z : Outport  Port=2
  wires:
  "phi "/1 -> Cos3/1
  Gravity/1 -> Display1/1, Z''/2
  Z''/1 -> Integrator/1
  Integrator1/1 -> z/1, Display2/1, Scope1/1
  "theta "/1 -> Cos2/1
  Integrator/1 -> dot_z/1, Integrator1/1
  Cos2/1 -> Product4/2
  Cos3/1 -> Product4/1
  T/1 -> T/m 2/1
  Product4/1 -> Product/1
  Product/1 -> Display/1, Z''/1
  T/m 2/1 -> Product/2
  Altitude Initial/1 -> Integrator1/2

== system model_for_testing_errors_2/Quadrotor System/Subsystem psi ==
  note: .
  note: \psi
  note: \psi
  note: \psi = q(S_\phi/C_\theta) + r(C_\phi/C_\theta) (4)
  note: .
  q : Inport
  r : Inport  Port=2
  phi : Inport  Port=3
  theta : Inport  Port=4
  Display1 : Display
  Display16 : Display
  Display17 : Display
  Divide : Product  Inputs=/
  Divide1 : Product  Inputs=/
  Integrator8 : Integrator  InitialConditionSource=external  InitialCondition=-pi
  Product10 : Product  Inputs=3
  Product9 : Product  Inputs=3
  Yaw Initial : Constant  Value=psi0
  Z''5 : Sum
  sin 3 : Trigonometry  Operator=cos
  sin 4 : Trigonometry  Operator=cos
  sin 5 : Trigonometry
  sin 6 : Trigonometry  Operator=cos
  psi : Outport
  wires:
  sin 3/1 -> Product9/1
  Divide1/1 -> Product10/3
  sin 5/1 -> Product10/1
  sin 4/1 -> Divide/1
  Divide/1 -> Product9/3
  sin 6/1 -> Divide1/1
  Product9/1 -> Display16/1, Z''5/1
  theta/1 -> sin 6/1, sin 4/1
  phi/1 -> sin 5/1, sin 3/1
  q/1 -> Product10/2
  r/1 -> Product9/2
  Z''5/1 -> Integrator8/1
  Product10/1 -> Display17/1, Z''5/2
  Integrator8/1 -> Display1/1, psi/1
  Yaw Initial/1 -> Integrator8/2

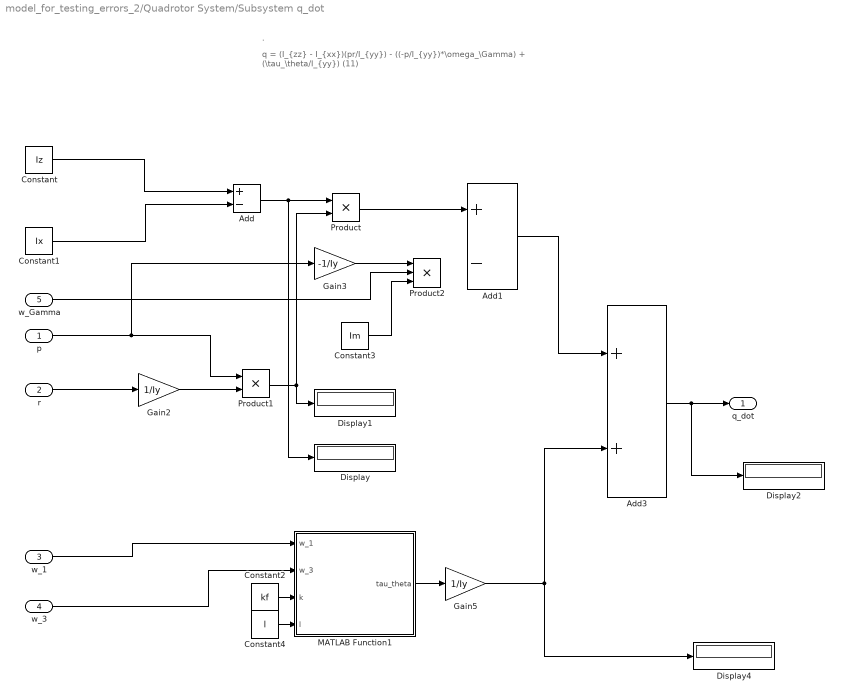
== system model_for_testing_errors_2/Quadrotor System/Subsystem q_dot ==
  note: q = (I_{zz} - I_{xx})(pr/I_{yy}) - ((-p/I_{yy})*\omega_\Gamma) + (\tau_\theta/I_{yy}) (11)
  note: .
  "p " : Inport
  r : Inport  Port=2
  w_1 : Inport  Port=3
  w_3 : Inport  Port=4
  "w_Gamma " : Inport  Port=5
  Add : Sum  Inputs=+-
  Add1 : Sum  Inputs=+-
  Add3 : Sum
  Constant : Constant  Value=Iz
  Constant1 : Constant  Value=Ix
  Constant2 : Constant  Value=kf
  Constant3 : Constant  Value=Im
  Constant4 : Constant  Value=l
  Display{,1..2,4} (4 alike) : Display
  Gain2 : Gain  Gain=1/Iy
  Gain3 : Gain  Gain=-1/Iy
  Gain5 : Gain  Gain=1/Iy
  MATLAB Function1 : MATLAB Function  TreatAsAtomicUnit=on
  Product : Product
  Product1 : Product
  Product2 : Product  Inputs=3
  q_dot : Outport
  wires:
  Constant/1 -> Add/1
  Constant1/1 -> Add/2
  Add/1 -> Display/1, Product/1
  Product1/1 -> Product/2, Display1/1
  Product/1 -> Add1/1
  Gain3/1 -> Product2/1
  r/1 -> Gain2/1
  Gain2/1 -> Product1/2
  "p "/1 -> Gain3/1, Product1/1
  w_3/1 -> MATLAB Function1/2(w_3)
  MATLAB Function1/1(tau_theta) -> Gain5/1
  w_1/1 -> MATLAB Function1/1(w_1)
  Add1/1 -> Add3/1
  Add3/1 -> q_dot/1, Display2/1
  "w_Gamma "/1 -> Product2/2
  Gain5/1 -> Display4/1, Add3/2
  Constant3/1 -> Product2/3
  Constant2/1 -> MATLAB Function1/3(k)
  Constant4/1 -> MATLAB Function1/4(l)

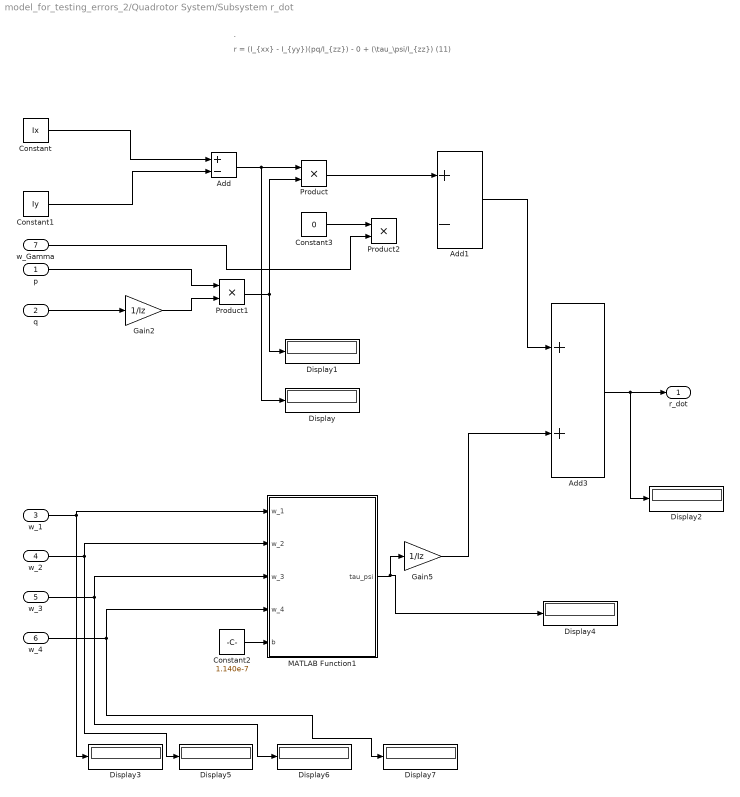
== system model_for_testing_errors_2/Quadrotor System/Subsystem r_dot ==
  note: r = (I_{xx} - I_{yy})(pq/I_{zz}) - 0 + (\tau_\psi/I_{zz}) (11)
  note: .
  "p " : Inport
  q : Inport  Port=2
  w_1 : Inport  Port=3
  w_2 : Inport  Port=4
  w_3 : Inport  Port=5
  w_4 : Inport  Port=6
  w_Gamma : Inport  Port=7
  Add : Sum  Inputs=+-
  Add1 : Sum  Inputs=+-
  Add3 : Sum
  Constant : Constant  Value=Ix
  Constant1 : Constant  Value=Iy
  Constant2 : Constant  Value=1.140e-7
  Constant3 : Constant  Value=0
  Display{,1..7} (8 alike) : Display
  Gain2 : Gain  Gain=1/Iz
  Gain5 : Gain  Gain=1/Iz
  MATLAB Function1 : MATLAB Function  TreatAsAtomicUnit=on
  Product : Product
  Product1 : Product
  Product2 : Product
  r_dot : Outport
  wires:
  Constant/1 -> Add/1
  Constant1/1 -> Add/2
  Add/1 -> Display/1, Product/1
  Product1/1 -> Display1/1, Product/2
  Product/1 -> Add1/1
  Constant3/1 -> Product2/1
  Add1/1 -> Add3/1
  Add3/1 -> Display2/1, r_dot/1
  "p "/1 -> Product1/1
  Gain2/1 -> Product1/2
  q/1 -> Gain2/1
  MATLAB Function1/1(tau_psi) -> Display4/1, Gain5/1
  w_1/1 -> MATLAB Function1/1(w_1), Display3/1
  w_2/1 -> MATLAB Function1/2(w_2), Display5/1
  w_4/1 -> MATLAB Function1/4(w_4), Display7/1
  w_Gamma/1 -> Product2/2
  Gain5/1 -> Add3/2
  w_3/1 -> MATLAB Function1/3(w_3), Display6/1
  Constant2/1 -> MATLAB Function1/5(b)

== system model_for_testing_errors_2/Quadrotor System/Subsystem theta ==
  note: \theta
  note: .
  note: \theta
  note: .
  note: \theta = q(C_\phi) - r(S_\theta) (4)
  q : Inport
  r : Inport  Port=2
  "phi " : Inport  Port=3
  Display1 : Display
  Display13 : Display
  Display14 : Display
  Integrator7 : Integrator  InitialConditionSource=external  InitialCondition=-0.09
  Pitch Initial : Constant  Value=0
  Product7 : Product
  Product8 : Product
  Z''4 : Sum  Inputs=-+
  sin 1 : Trigonometry  Operator=cos
  sin 2 : Trigonometry
  theta : Outport
  wires:
  "phi "/1 -> sin 1/1, sin 2/1
  r/1 -> Product7/2
  sin 1/1 -> Product8/1
  Product8/1 -> Display14/1, Z''4/2
  Z''4/1 -> Integrator7/1
  sin 2/1 -> Product7/1
  Product7/1 -> Display13/1, Z''4/1
  q/1 -> Product8/2
  Integrator7/1 -> Display1/1, theta/1
  Pitch Initial/1 -> Integrator7/2

== system model_for_testing_errors_2/linear motion/Subsystem ==
  T : Inport
  theta : Inport  Port=2
  phi : Inport  Port=3
  (F_ind+F_flap+F_drag)_z : Inport  Port=4
  Constant4 : Constant  Value=m*g
  Cos4 : Trigonometry  Operator=cos
  Cos5 : Trigonometry  Operator=cos
  Gain4 : Gain  Gain=1/m
  Product2 : Product  Inputs=3
  Sum2 : Sum  Inputs=|+--
  ddot_r_z : Outport
  wires:
  Product2/1 -> Sum2/1
  phi/1 -> Cos4/1
  theta/1 -> Cos5/1
  T/1 -> Product2/1
  Cos4/1 -> Product2/2
  Constant4/1 -> Sum2/3
  Cos5/1 -> Product2/3
  (F_ind+F_flap+F_drag)_z/1 -> Sum2/2
  Sum2/1 -> Gain4/1
  Gain4/1 -> ddot_r_z/1  "ddot_r_z"

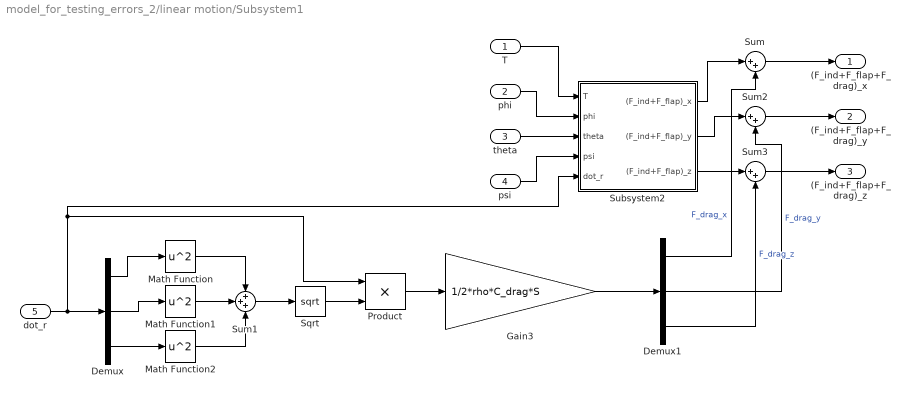
== system model_for_testing_errors_2/linear motion/Subsystem1 ==
  T : Inport
  phi : Inport  Port=2
  theta : Inport  Port=3
  psi : Inport  Port=4
  dot_r : Inport  Port=5
  Demux : Demux  Outputs=3
  Demux1 : Demux  Outputs=3
  Gain3 : Gain  Gain=1/2*rho*C_drag*S
  Math Function : Math  Operator=square
  Math Function1 : Math  Operator=square
  Math Function2 : Math  Operator=square
  Product : Product
  Sqrt : Sqrt
  Subsystem2 : Subsystem
  Sum : Sum  Inputs=|++
  Sum1 : Sum  Inputs=+++
  Sum2 : Sum  Inputs=|++
  Sum3 : Sum  Inputs=|++
  (F_ind+F_flap+F_drag)_x : Outport
  (F_ind+F_flap+F_drag)_y : Outport  Port=2
  (F_ind+F_flap+F_drag)_z : Outport  Port=3
  wires:
  Demux1/2 -> Sum2/2  "F_drag_y"
  dot_r/1 -> Product/1, Subsystem2/5(dot_r), Demux/1
  Math Function1/1 -> Sum1/2
  Demux/1 -> Math Function/1
  Demux/2 -> Math Function1/1
  Sum1/1 -> Sqrt/1
  Math Function/1 -> Sum1/1
  Demux/3 -> Math Function2/1
  Demux1/3 -> Sum3/2  "F_drag_z"
  Subsystem2/2((F_ind+F_flap)_y) -> Sum2/1
  Math Function2/1 -> Sum1/3
  Sqrt/1 -> Product/2
  phi/1 -> Subsystem2/2(phi)
  Product/1 -> Gain3/1
  T/1 -> Subsystem2/1(T)
  theta/1 -> Subsystem2/3(theta)
  psi/1 -> Subsystem2/4(psi)
  Gain3/1 -> Demux1/1
  Subsystem2/1((F_ind+F_flap)_x) -> Sum/1
  Subsystem2/3((F_ind+F_flap)_z) -> Sum3/1
  Demux1/1 -> Sum/2  "F_drag_x"
  Sum/1 -> (F_ind+F_flap+F_drag)_x/1
  Sum2/1 -> (F_ind+F_flap+F_drag)_y/1
  Sum3/1 -> (F_ind+F_flap+F_drag)_z/1

== system model_for_testing_errors_2/linear motion/Subsystem2 ==
  psi : Inport
  T : Inport  Port=2
  theta : Inport  Port=3
  phi : Inport  Port=4
  (F_ind+F_flap+F_drag)_y : Inport  Port=5
  Cos2 : Trigonometry  Operator=cos
  Cos3 : Trigonometry
  Cos6 : Trigonometry
  Cos7 : Trigonometry
  Cos8 : Trigonometry  Operator=cos
  Gain3 : Gain  Gain=1/m
  Product1 : Product
  Product3 : Product
  Product4 : Product  Inputs=3
  Sum1 : Sum  Inputs=|+-
  Sum3 : Sum  Inputs=|+-
  ddot_r_y : Outport
  wires:
  Cos6/1 -> Product4/1
  theta/1 -> Cos6/1
  psi/1 -> Cos7/1, Cos2/1
  Cos7/1 -> Product4/2
  Sum1/1 -> Gain3/1
  phi/1 -> Cos8/1, Cos3/1
  Cos8/1 -> Product4/3
  Cos2/1 -> Product3/1
  Cos3/1 -> Product3/2
  Product4/1 -> Sum3/1
  Product3/1 -> Sum3/2
  T/1 -> Product1/1
  Sum3/1 -> Product1/2
  Product1/1 -> Sum1/1
  (F_ind+F_flap+F_drag)_y/1 -> Sum1/2
  Gain3/1 -> ddot_r_y/1  "ddot_r_y"
